simulink model "ADRC_DaoLiBai_test2"  (R2018b)
settings: Solver=VariableStepAuto  StartTime=0.0  StopTime=10  RelTol=1e-3
settings Model: Creator=ILQMN  LastModifiedBy=ILQMN

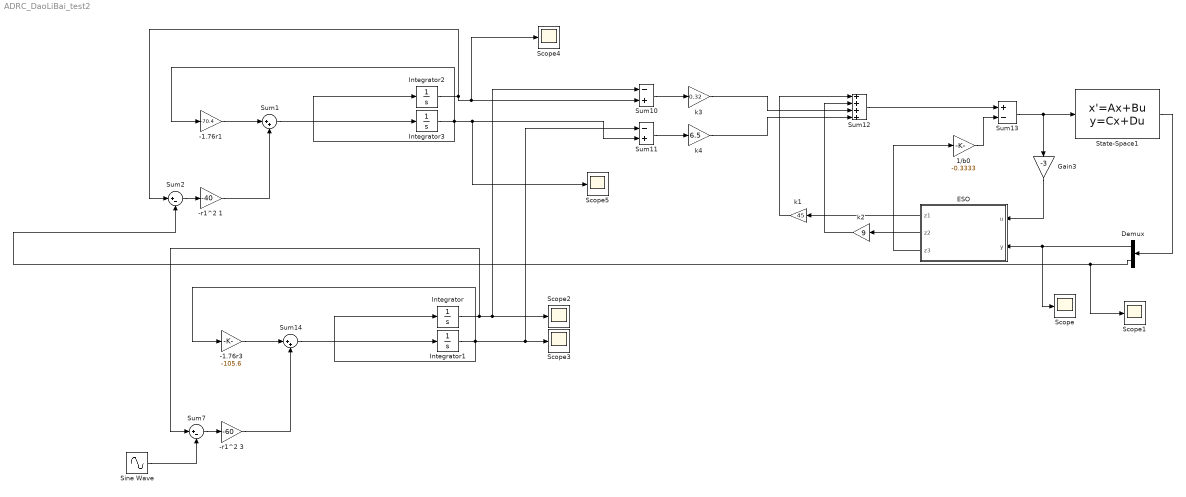
== system ADRC_DaoLiBai_test2 ==
  -1.76r1 : Gain  Gain=-70.4
  -1.76r3 : Gain  Gain=-105.6
  -r1^2 1 : Gain  Gain=-40
  -r1^2 3 : Gain  Gain=-60
  "1/b0 " : Gain  Gain=-0.3333
  Demux : Demux  Outputs=2
  ESO : Subsystem
  Gain3 : Gain  Gain=-3
  Integrator{,1..3} (4 alike) : Integrator
  Scope{,1..5} (6 alike) : Scope
  Sine Wave : Sin  SampleTime=0
  State-Space1 : StateSpace  A=[0 1 0 0;27.828 0 0 -0.2357;0 0 0 1;0.6393 0 0 -0.08832]  B=[0;2.6683;0;0.8832]  C=[1 0 0 0;0 0 1 0]  D=[0;0]  InitialCondition=[0;0;0;0]
  Sum1 : Sum  Inputs=|++
  Sum10 : Sum  Inputs=-+
  Sum11 : Sum  Inputs=-+
  Sum12 : Sum  Inputs=++++
  Sum13 : Sum  Inputs=+-
  Sum14 : Sum  Inputs=|++
  Sum2 : Sum  Inputs=|+-
  Sum7 : Sum  Inputs=|+-
  k1 : Gain  Gain=45
  k2 : Gain  Gain=9
  k3 : Gain  Gain=0.32
  "k4 " : Gain  Gain=6.5
  wires:
  Integrator/1 -> Sum10/1, Scope2/1, Sum7/1
  Sum14/1 -> Integrator1/1
  -1.76r3/1 -> Sum14/1
  Sum7/1 -> -r1^2 3/1
  -r1^2 3/1 -> Sum14/2
  Gain3/1 -> ESO/1("u ")
  Integrator1/1 -> Sum11/1, Scope3/1, Integrator/1, -1.76r3/1
  k3/1 -> Sum12/3
  ESO/1(z1) -> k1/1
  ESO/2(z2) -> k2/1
  "k4 "/1 -> Sum12/4
  State-Space1/1 -> Demux/1
  Sine Wave/1 -> Sum7/2
  k2/1 -> Sum12/2
  "1/b0 "/1 -> Sum13/2
  Sum10/1 -> k3/1
  Sum13/1 -> State-Space1/1, Gain3/1
  Demux/1 -> Scope/1, ESO/2("y ")
  Sum12/1 -> Sum13/1
  k1/1 -> Sum12/1
  Sum11/1 -> "k4 "/1
  Demux/2 -> Sum2/2, Scope1/1
  Integrator2/1 -> Scope4/1, Sum10/2, Sum2/1
  -r1^2 1/1 -> Sum1/2
  Sum2/1 -> -r1^2 1/1
  -1.76r1/1 -> Sum1/1
  Integrator3/1 -> Integrator2/1, Scope5/1, Sum11/2, -1.76r1/1
  Sum1/1 -> Integrator3/1
  ESO/3(z3) -> "1/b0 "/1

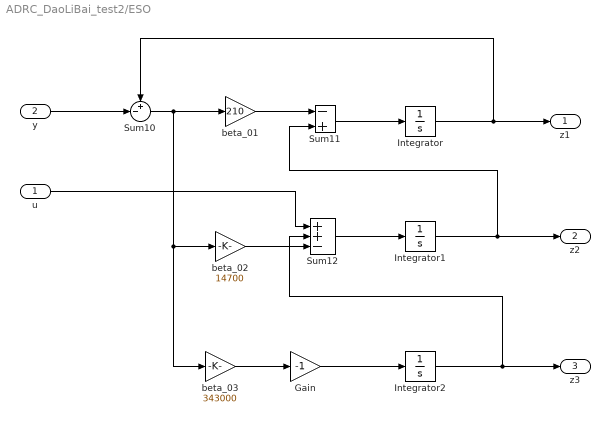
== system ADRC_DaoLiBai_test2/ESO ==
  "u " : Inport
  "y " : Inport  Port=2
  Gain : Gain  Gain=-1
  Integrator : Integrator
  Integrator1 : Integrator
  Integrator2 : Integrator
  Sum10 : Sum  Inputs=+-|
  Sum11 : Sum  Inputs=-+
  Sum12 : Sum  Inputs=++-
  beta_01 : Gain  Gain=210
  beta_02 : Gain  Gain=14700
  beta_03 : Gain  Gain=343000
  z1 : Outport
  z2 : Outport  Port=2
  z3 : Outport  Port=3
  wires:
  beta_02/1 -> Sum12/3
  Gain/1 -> Integrator2/1
  Integrator1/1 -> Sum11/2, z2/1
  Integrator2/1 -> Sum12/2, z3/1
  Sum12/1 -> Integrator1/1
  "u "/1 -> Sum12/1
  beta_01/1 -> Sum11/1
  Sum10/1 -> beta_03/1, beta_02/1, beta_01/1
  Sum11/1 -> Integrator/1
  "y "/1 -> Sum10/2
  beta_03/1 -> Gain/1
  Integrator/1 -> z1/1, Sum10/1
